simulink model "ModeleNonLineaire"  (R2014b)
settings: Solver=ode45  StartTime=0.0  StopTime=10.0  RelTol=1e-3
values from neighbouring files (symbols this model uses):
  be1 = 13.029359254409743    (= 13.0293592544)    [Lissage_actionneur.m]
  g = 9.81    [bancEssaiConstantes.m]
  Jx = 1169e-06    (= 0.001169)    [bancEssaiConstantes.m]
  LA = LL    (= 0.115)    [bancEssaiConstantes.m]
  LB = LL    (= 0.115)    [bancEssaiConstantes.m]
  LC = LL    (= 0.115)    [bancEssaiConstantes.m]
  mP = 425e-03    (= 0.425)    [bancEssaiConstantes.m]
  mS = 0.0080    (= 0.008)    [bancEssaiConstantes.m]
  RA = RR    (= 3.6)    [bancEssaiConstantes.m]
  RB = RR    (= 3.6)    [bancEssaiConstantes.m]
  RC = RR    (= 3.6)    [bancEssaiConstantes.m]
  XA = +rABC    (= 0.0952)    [bancEssaiConstantes.m]
  XB = -rABC*sind(30)    [bancEssaiConstantes.m]
  XC = -rABC*sind(30)    [bancEssaiConstantes.m]
  XD = +rDEF*sind(30)    [bancEssaiConstantes.m]
  XE = -rDEF    (= -0.08)    [bancEssaiConstantes.m]
  XF = +rDEF*sind(30)    [bancEssaiConstantes.m]
  YA = 0.0    (= 0)    [bancEssaiConstantes.m]
  YB = +rABC*cosd(30)    [bancEssaiConstantes.m]
  YC = -rABC*cosd(30)    [bancEssaiConstantes.m]
  YD = +rDEF*cosd(30)    [bancEssaiConstantes.m]
  YE = 0.0    (= 0)    [bancEssaiConstantes.m]
  YF = -rDEF*cosd(30)    [bancEssaiConstantes.m]
undefined symbols (not defined in the file or in its folder): ae0, ae1, ae2, ae3, as0, as1, as2, as3, VA, VB, VC
settings Model: Creator=godj2407  LastModifiedBy=godj2407

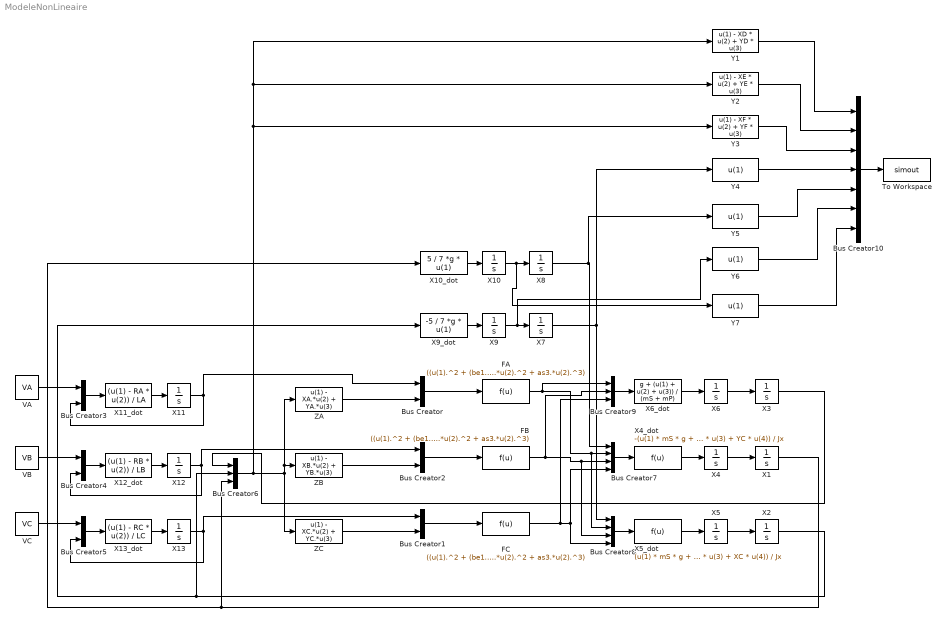
== system ModeleNonLineaire ==
  Bus Creator{,1..5} (6 alike) : BusCreator  Inputs=2
  Bus Creator10 : BusCreator  Inputs=7
  Bus Creator6 : BusCreator  Inputs=3
  Bus Creator7 : BusCreator
  Bus Creator8 : BusCreator
  Bus Creator9 : BusCreator  Inputs=3
  "FA " : Fcn  Tag=FA  Expr=((u(1).^2 + (be1.*abs(u(1)))).*sign(u(1)))./(ae0 + ae1.*u(2) + ae2.*u(2).^2 + ae3.*u(2).^3) + (-1)./(as0 + as1.*u(2) + as2.*u(2).^2 + as3.*u(2).^3)
  FB : Fcn  Tag=FA  Expr=((u(1).^2 + (be1.*abs(u(1)))).*sign(u(1)))./(ae0 + ae1.*u(2) + ae2.*u(2).^2 + ae3.*u(2).^3) + (-1)./(as0 + as1.*u(2) + as2.*u(2).^2 + as3.*u(2).^3)
  FC : Fcn  Tag=FA  Expr=((u(1).^2 + (be1.*abs(u(1)))).*sign(u(1)))./(ae0 + ae1.*u(2) + ae2.*u(2).^2 + ae3.*u(2).^3) + (-1)./(as0 + as1.*u(2) + as2.*u(2).^2 + as3.*u(2).^3)
  To Workspace : ToWorkspace  VariableName=simout  SaveFormat=Timeseries  SampleTime=-1
  VA : Constant  Value=VA
  VB : Constant  Value=VB
  VC : Constant  Value=VC
  X{1..3,5..13} (12 alike) : Integrator
  X10_dot : Fcn  Tag=FA  Expr=5 / 7 *g * u(1)
  X11_dot : Fcn  Expr=(u(1) - RA * u(2)) / LA
  X12_dot : Fcn  Expr=(u(1) - RB * u(2)) / LB
  X13_dot : Fcn  Expr=(u(1) - RC * u(2)) / LC
  "X4 " : Integrator
  X4_dot : Fcn  Tag=FA  Expr=-(u(1) * mS * g + YA * u(2) + YB * u(3) + YC * u(4)) / Jx
  X5_dot : Fcn  Tag=FA  Expr=(u(1) * mS * g + XA * u(2) + XB * u(3) + XC * u(4)) / Jx
  X6_dot : Fcn  Tag=FA  Expr=g + (u(1) + u(2) + u(3)) / (mS + mP)
  X9_dot : Fcn  Tag=FA  Expr=-5 / 7 *g * u(1)
  Y1 : Fcn  Tag=FA  Expr=u(1) - XD * u(2) + YD * u(3)
  Y2 : Fcn  Tag=FA  Expr=u(1) - XE * u(2) + YE * u(3)
  Y3 : Fcn  Tag=FA  Expr=u(1) - XF * u(2) + YF * u(3)
  Y{4..7} (4 alike) : Fcn  Tag=FA  Expr=u(1)
  "ZA " : Fcn  Expr=u(1) - XA.*u(2) + YA.*u(3)
  "ZB " : Fcn  Expr=u(1) - XB.*u(2) + YB.*u(3)
  "ZC " : Fcn  Expr=u(1) - XC.*u(2) + YC.*u(3)
  wires:
  Bus Creator/1 -> "FA "/1
  "ZA "/1 -> Bus Creator/2
  Bus Creator2/1 -> FB/1
  "ZB "/1 -> Bus Creator2/2
  "ZC "/1 -> Bus Creator1/2
  Bus Creator1/1 -> FC/1
  X11_dot/1 -> X11/1
  Bus Creator3/1 -> X11_dot/1
  X11/1 -> Bus Creator3/2, Bus Creator/1
  VA/1 -> Bus Creator3/1
  X12_dot/1 -> X12/1
  Bus Creator4/1 -> X12_dot/1
  X12/1 -> Bus Creator2/1, Bus Creator4/2
  VB/1 -> Bus Creator4/1
  X13_dot/1 -> X13/1
  Bus Creator5/1 -> X13_dot/1
  X13/1 -> Bus Creator5/2, Bus Creator1/1
  VC/1 -> Bus Creator5/1
  X4_dot/1 -> "X4 "/1
  Bus Creator6/1 -> Y1/1, Y2/1, Y3/1, "ZA "/1, "ZB "/1, "ZC "/1
  "X4 "/1 -> X1/1
  Bus Creator7/1 -> X4_dot/1
  FB/1 -> Bus Creator9/2, Bus Creator8/3, Bus Creator7/3
  "FA "/1 -> Bus Creator9/1, Bus Creator8/2, Bus Creator7/2
  FC/1 -> Bus Creator9/3, Bus Creator7/4, Bus Creator8/4
  X5_dot/1 -> X5/1
  Bus Creator8/1 -> X5_dot/1
  X5/1 -> X2/1
  X6_dot/1 -> X6/1
  Bus Creator9/1 -> X6_dot/1
  X6/1 -> X3/1
  X9_dot/1 -> X9/1
  X9/1 -> Y6/1, X7/1
  X7/1 -> Y4/1, Bus Creator8/1
  X2/1 -> Bus Creator6/2, X9_dot/1
  X10_dot/1 -> X10/1
  X10/1 -> Y7/1, X8/1
  X3/1 -> Bus Creator6/1
  X1/1 -> X10_dot/1, Bus Creator6/3
  X8/1 -> Y5/1, Bus Creator7/1
  Y4/1 -> Bus Creator10/4
  Y3/1 -> Bus Creator10/3
  Y2/1 -> Bus Creator10/2
  Y1/1 -> Bus Creator10/1
  Y5/1 -> Bus Creator10/5
  Y6/1 -> Bus Creator10/6
  Y7/1 -> Bus Creator10/7
  Bus Creator10/1 -> To Workspace/1
